simulink model "CM13_2024a_MachE_for_UA_HIL"  (R2024a)
settings: Solver=ode1  StartTime=0.0  StopTime=Inf  FixedStep=0.001  RelTol=1e-3  EnableMultiTasking=on
PreLoadFcn:
  | % if ~length(which('cmcmd')), cmenv; end
PostLoadFcn:
  | if any(exist('dsrtsu_mdlpostloadfcn', 'file') ~= 0), dsrtsu_mdlpostloadfcn('Execute', bdroot); end
InitFcn:
  | , if any(exist('rtifpga_mdlclblib', 'file') ~= 0), rtifpga_mdlclblib('Init', bdroot); end,
  | , if any(exist('dsmpb_private', 'file') ~= 0), dsmpb_private('dsmpb_mdlclblib', 'Init', bdroot); end,
values from neighbouring files (symbols this model uses):
  CoastDown =     [Run_Simulink.mat]
  limitedMCT =     [Run_Simulink.mat]
  MCT =     [Run_Simulink.mat]
  pMCT =     [Run_Simulink.mat]
  RealSimPara =     [Run_Simulink.mat]
  Ref_speed = [13 13.007895099 13.015778396 13.023649891 13.031509584 13.039357475 13.047193564 13.055017851 13.062830336 13.070631019 13.0784199 13.086196979 ... (2669 elements, 2669x1)]    [Ref_speed_and_time.mat]
  Ref_time = [0 0.01 0.02 0.03 0.04 0.05 0.06 0.07 0.08 0.09 0.1 0.11 ... (2669 elements, 2669x1)]    [Ref_speed_and_time.mat]
  US06 =     [Run_Simulink.mat]
undefined symbols (not defined in the file or in its folder): AccelCmd, ActTqLF_Nm_, ActTqLR_Nm_, ActTqRF_Nm_, ActTqRR_Nm_, BattChargeLimitMaxPwr, BattChargeLimitSocBpts, BattChargeLimitTbl, BattChrgCapcty, BattDischargeLimitSocBpts, BattDischargeLimitTbl, BattDischargeMaxPwr, BattNumCellsParallel, BattNumCellsSeries, BattOpenVoltCapBpts, BattOpenVoltTbl, BattResistSocBpts, BattResistTbl, BattResistTempBpts, BrakeMaxPrs, BrakeMaxTrq, ChassisDistCg2FrontAxle, ChassisDistCg2RearAxle, ChassisVehMass, CltchCmd, DecelCmd, DiffRatio, DiscIntNeverNeededParam, EnvGravCnst, EnvPrs, EnvTemp, FuelSpecificGrav, GearCmd, h, InitStates, lgSw, MtrEffSpdBpts, MtrEffTbl, MtrEffTrqBpts, MtrPwrMax, MtrTrqMax, planned_speed, planned_time, ref_speed, ref_time, rticanmm_blockfcn, rticanmm_initfcn, SteeringCmd, SupvsryCtrlRegenBrkCutOffTbl, SupvsryCtrlRegenSpdBpts, TestScnrioCycleNum, VEH
libraries: simulink x264, VSIGenLib x262, etargetslib x201, dsmpblib x161, CarMaker4SL x142, rtimmsu_dsrtlib x32, vehdynlibtire x24, autolibshared x19, vehdynlibsuspension x14, vehdynlibtirecommon x14, autolibutils x10, VsrLibWheel x8
(part 48 of 48)

== matlab function CM13_2024a_MachE_for_UA_HIL/RealSim1/MATLAB Function3 ==
  data: simState input; connectionState input; timeSimulator input; timeStepSimulator output; timeStepSimulatorPrevious input; timeStepTrigger output
function [timeStepSimulator, timeStepTrigger]  = fcn(simState, connectionState, timeSimulator, timeStepSimulatorPrevious)


if simState && abs(connectionState-3) < 1e-5 && (timeSimulator >= timeStepSimulatorPrevious + 0.1 - 1e-5 || abs(timeSimulator) < 1e-5)
    timeStepSimulator = timeSimulator;
    timeStepTrigger = 1;
else
    timeStepSimulator = timeStepSimulatorPrevious;
    timeStepTrigger = 0;
end

== matlab function CM13_2024a_MachE_for_UA_HIL/RealSim1/MATLAB Function4 ==
  data: simState input; simulatorStartTime output; simStatePrevious input; connectionState input; simulationTime input; simState output
function [simulatorStartTime, simState] = fcn(simState, simStatePrevious, connectionState, simulationTime)


if abs(simState - 1) < 1e-5 && abs(simStatePrevious) < 1e-5 && abs(connectionState-3) < 1e-5
    % set connectionState and start time
    simulatorStartTime = simulationTime;
else
    simulatorStartTime = 0;
end

== matlab function CM13_2024a_MachE_for_UA_HIL/FIXS1/RealSim Core/MATLAB Function1 ==
  data: obj input; simState output; ByteData input; nByte input; connectionState input; t output; nVeh output; VehDataBus output; isVehicleInNetwork output
function [simState, t, nVeh, VehDataBus, isVehicleInNetwork] = stepImpl(obj, ByteData, nByte, connectionState)

    simState = obj.simStatePrevious;
    t = obj.tPrevious;
    nVeh = 0;
    
    % init values for other variables
    totalMsgSize = 0; % this is the total message size received from Real-Sim
    msgProcessed = 0; % to record how many messages have been processed
    
    VehDataBus = obj.VehicleDataPrevious;

    %---------------------------
    % read received buffer
    %---------------------------
    % need to check size, before connection, there could be no
    % message at all             
    if nByte >= obj.msgHeaderSize
        simState = double(typecast(uint8(ByteData(1)),'uint8'));
        t = double(typecast(uint8(ByteData(2:5)),'single'));
        totalMsgSize = double(typecast(uint8(ByteData(6:9)),'uint32'));
        msgProcessed = obj.msgHeaderSize;
        
        obj.simStatePrevious = simState;
        obj.tPrevious = t;
    end
    
    % read actual message fields
    while round(msgProcessed) < round(totalMsgSize)
        iMsgSizeRecv = double(typecast(uint8(ByteData(msgProcessed+1:msgProcessed+2)),'uint16'));
        iMsgTypeRecv = double(typecast(uint8(ByteData(msgProcessed+3)),'uint8'));

        % !!! for now, Simulink only supports vehicle data type
        if obj.enableDebug
            obj.vehMsgIdentifer = iMsgTypeRecv;
        else
            obj.vehMsgIdentifer = 1;
        end
        
        if iMsgTypeRecv == obj.vehMsgIdentifer
            VehDataBus = obj.depackVehData(VehDataBus, ByteData(msgProcessed+obj.msgEachHeaderSize+1:msgProcessed+iMsgSizeRecv));
               
            nVeh = nVeh + 1;

            obj.VehicleDataPrevious = VehDataBus;
            obj.isVehicleInNetworkPrevious = 1;
        else
            % not supported yet!!!
            
        end
        
        msgProcessed = msgProcessed + iMsgSizeRecv;

    end
    

    if abs(connectionState-3)>1e-5
        % if not connected, then set to 0
        obj.simStatePrevious = 0;
        obj.tPrevious = 0;
        obj.nVehPrevious = 0;
        obj.VehicleDataPrevious = obj.VehicleDataEmpty;
        obj.isVehicleInNetworkPrevious = 0;
    else
        if totalMsgSize == 9
            obj.isVehicleInNetworkPrevious = 0;
        end
    end
    isVehicleInNetwork = obj.isVehicleInNetworkPrevious;

== matlab function CM13_2024a_MachE_for_UA_HIL/FIXS1/RealSim Core/generateTimeStepTrigger ==
  data: simState input; connectionState input; timeSimulation input; timeSimulationOut output; timeInOut output; timeSimulationPrevious input; timeStepTrigger output; timeIn input; timeInPrevious input
function [timeSimulationOut, timeInOut, timeStepTrigger]  = fcn(simState, connectionState, timeSimulation, timeSimulationPrevious, timeIn, timeInPrevious)


%if simState && abs(connectionState-3) < 1e-5 && (timeSimulator >= timeStepSimulatorPrevious + 0.1 - 1e-5 || abs(timeSimulator) < 1e-5)
% if simState && abs(connectionState-3) < 1e-5 && (timeSimulation >= timeSimulationPrevious + 0.1 - 1e-5)
if simState && abs(connectionState-3) < 1e-5 && ((timeSimulation >= timeSimulationPrevious + 0.1 - 1e-5) && (timeIn >= timeInPrevious + 0.1 - 1e-5))
    timeSimulationOut = timeSimulation;
    timeInOut = timeIn;
    timeStepTrigger = 1;
else
    timeSimulationOut = timeSimulationPrevious;
    timeInOut = timeInPrevious;
    timeStepTrigger = 0;
end

== matlab function CM13_2024a_MachE_for_UA_HIL/FIXS1/RealSim Translate CM Signal to Bus as Feedback to SUMO//VISSIM/MATLAB Function ==
  data: CM_POI_X input; positionX output; positionY output; positionZ output; heading output; color output; speedDesired output; CM_POI_Y input; CM_POI_Z input; CM_Fr1_X input; CM_Fr1_Y input; CM_Fr1_Z input; CM_yaw input; color_rgba input; CM_speed input
function [positionX, positionY, positionZ, heading, color, speedDesired] = ...
    RealSimSigTrans(CM_POI_X, CM_POI_Y, CM_POI_Z, CM_Fr1_X, CM_Fr1_Y, CM_Fr1_Z, CM_yaw, color_rgba, CM_speed)

% intialization
positionX = 0;
positionY = 0;
positionZ = 0;
heading = 0;
color = 0;
speedDesired = 0;

% convert position
% CM POI is CoM, CM Fr1 is back bottom of car
% SUMO-xy is front of car
% SUMO-z is bottom of car
positionX = CM_POI_X + (CM_POI_X - CM_Fr1_X);
positionY = CM_POI_Y + (CM_POI_Y - CM_Fr1_Y);
positionZ = CM_Fr1_Z;

% convert heading
if (CM_yaw >= -pi && CM_yaw <= 0.5 * pi)
    heading = ((-CM_yaw + 0.5 * pi) * 180 / pi);
else
    heading = ((-CM_yaw + 2.5 * pi) * 180 / pi);
end

% convert color from rgba to uint32
color = sum(color_rgba.*[2^24;2^16;2^8;2^0]);

% speed is same unit
speedDesired = CM_speed;

== stateflow chart CM13_2024a_MachE_for_UA_HIL/FIXS1/RealSimHILCycle ==
  state CycleOn
    state InitialWait
      CycleMode=1;
    state RampUp
      CycleMode=2;
      SpeedCmd=SpeedCmd+0.1
    state Driving
      CycleMode=3;
      SpeedCmd=max(SpeedIn, 0)
    state WaitForNextRamp
    InitialWait -> RampUp : [after(InitWaitTime,sec) || RampUpFlag]
    (default) -> InitialWait
    RampUp -> Driving [order 1] : [abs(SpeedCmd-SpeedInit)<0.5]
    RampUp -> CycleOn.WaitForNextRamp [order 2] : [abs(SpeedCmd-SpeedInit)>=0.1]
    CycleOn.WaitForNextRamp -> RampUp : after(0.1,sec)
  state Idle
    CycleMode=0;
    SpeedCmd=0;
    CycleTime=0;
  state RampDown
    CycleMode=4;
    SpeedCmd=SpeedCmd-1;
  state WaitForNextRamp
  (default) -> Idle
  Idle -> CycleOn : [SimState>=6 && ...
      | DistanceTravel <= totalDistance && ...
      | SimTime <= totalTime && ...
      | ~RampDownFlag]
  RampDown -> Idle [order 1] : [SpeedCmd<0.5]
  CycleOn -> RampDown : [DistanceTravel > totalDistance || ...
      | SimTime > totalTime || ...
      | RampDownFlag || ...
      | SimState==9]
  WaitForNextRamp -> RampDown : after(0.1,sec)
  RampDown -> WaitForNextRamp [order 2] : [SpeedCmd>=0.5]
  data: SimTime input; SimState input; SpeedIn input; DistanceTravel input; InitWaitTime input; SpeedInit input; totalDistance input; CycleMode output; SpeedCmd output; totalTime input; RampDownFlag input; CycleTime local; RampUpFlag input

== matlab function CM13_2024a_MachE_for_UA_HIL/RealSim2/MATLAB Function ==
  data: strUint8Vec input; intVal output double; strLen input
function intVal = strVec2Int(strUint8Vec, strLen)

    strVec = blanks(50);
    for i = 1:strLen
       strVec(i) = strUint8Vec(i); 
    end
    if strLen > 0
        intVal = real(str2double(strVec(1:strLen)));
    else
        intVal = -1;
    end

== matlab function CM13_2024a_MachE_for_UA_HIL/RealSim2/MATLAB Function1 ==
  data: strUint8Vec input; intVal output double; strLen input
function intVal = strVec2Int(strUint8Vec, strLen)

    strVec = blanks(50);
    for i = 1:strLen
       strVec(i) = strUint8Vec(i); 
    end
    if strLen > 0
        intVal = real(str2double(strVec(1:strLen)));
    else
        intVal = -1;
    end

== matlab function CM13_2024a_MachE_for_UA_HIL/RealSim2/MATLAB Function2 ==
  data: signalLightId input uint8 size=[1 50]; signalLightIdString output string; signalLightIdLength input
function signalLightIdString = fcn(signalLightId, signalLightIdLength)

signalLightIdString = string(char(signalLightId));

== matlab function CM13_2024a_MachE_for_UA_HIL/RealSim2/MATLAB Function3 ==
  data: simState input; connectionState input; timeSimulator input; timeStepSimulator output; timeStepSimulatorPrevious input; timeStepTrigger output
function [timeStepSimulator, timeStepTrigger]  = fcn(simState, connectionState, timeSimulator, timeStepSimulatorPrevious)


if simState && abs(connectionState-3) < 1e-5 && (timeSimulator >= timeStepSimulatorPrevious + 0.1 - 1e-5 || abs(timeSimulator) < 1e-5)
    timeStepSimulator = timeSimulator;
    timeStepTrigger = 1;
else
    timeStepSimulator = timeStepSimulatorPrevious;
    timeStepTrigger = 0;
end

== matlab function CM13_2024a_MachE_for_UA_HIL/RealSim2/MATLAB Function4 ==
  data: simState input; simulatorStartTime output; simStatePrevious input; connectionState input; simulationTime input; simState output
function [simulatorStartTime, simState] = fcn(simState, simStatePrevious, connectionState, simulationTime)


if abs(simState - 1) < 1e-5 && abs(simStatePrevious) < 1e-5 && abs(connectionState-3) < 1e-5
    % set connectionState and start time
    simulatorStartTime = simulationTime;
else
    simulatorStartTime = 0;
end

== stateflow chart CM13_2024a_MachE_for_UA_HIL/Vehicle Under Test2/Vehicle/Actuation and Outputs/MOOG Brake Actuator/MOOG Interface/MOOG State Machine ==
  state MainStateMachine [parallel]
    settings: executionOrder=2
    state Learning
      state LearnMinStop
        en:
        state BackStopCmd
          en:
          MoogOpMode=21 ;
          PositionCmd=-100000;
        state BackStopReached
          en:
          MoogOpMode=22;
          PositionCmd=0;
        state BackStopSettle
          en:
          MoogOpMode=23;
          MinStop=ActualPosition_cnt;
          PositionCmd=0;
        (default) -> MainStateMachine.Learning.LearnMinStop.BackStopCmd
        MainStateMachine.Learning.LearnMinStop.BackStopCmd -> MainStateMachine.Learning.LearnMinStop.BackStopReached : [bitand(StatusWord,8)]
        MainStateMachine.Learning.LearnMinStop.BackStopReached -> MainStateMachine.Learning.LearnMinStop.BackStopSettle : after(2,sec)
      state StartLearning
        en:
        MoogOpMode=11;
        PositionCmd=0;
        MinStop=-200000;
        MaxStop=200000;
      state LearnMaxStop
        en:
        state BackStopCmd
          en:
          MoogOpMode=31;
          PositionCmd=100000;
        state BackStopReached
          en:
          MoogOpMode=32;
          PositionCmd=0;
        state BackStopSettle
          en:
          MoogOpMode=33;
          MaxStop=ActualPosition_cnt;
          PositionCmd=0;
        (default) -> MainStateMachine.Learning.LearnMaxStop.BackStopCmd
        MainStateMachine.Learning.LearnMaxStop.BackStopCmd -> MainStateMachine.Learning.LearnMaxStop.BackStopReached : [bitand(StatusWord,8)]
        MainStateMachine.Learning.LearnMaxStop.BackStopReached -> MainStateMachine.Learning.LearnMaxStop.BackStopSettle : after(2,sec)
      state EndLearning
        en:
        MoogOpMode=41;
        PositionCmd=0;
        LearningComplete=1;
        FaultCntr=0;
      (default) -> StartLearning
      StartLearning -> LearnMinStop : after(0.5,sec)[InitComplete ==1]
      LearnMinStop -> LearnMaxStop : after(1,sec)[InitComplete ==1  && MinStop ~=-200000]
      LearnMaxStop -> EndLearning : after(1,sec)[InitComplete ==1  && MaxStop ~=200000 && ((MaxStop-MinStop)>ActuatorMinTravelForReady)]
    state NormalOperation
      state LearningNotComplete
        en:
        MoogOpMode=101;
        Actuator_Ready=0;
        du:
        PositionCmd=0;
      state LearningComplete
        en:
        MoogOpMode=102;
        Actuator_Ready=1;
        du:
        PositionCmd=TargetPosition_cnt;
      (default) -> LearningNotComplete
      LearningNotComplete -> LearningComplete : after(1,sec)[LearningComplete==1]
    MainStateMachine.Learning.LearnMaxStop.BackStopSettle -> NormalOperation : after(10,sec)
    Learning -> NormalOperation : after(1,sec)[LearningComplete==1]
    NormalOperation -> Learning : [PositionLearningTrigger==1]{Actuator_Ready =0;
        | LearningComplete=0}
    (default) -> NormalOperation : {Actuator_Ready =0;
        | LearningComplete=0}
  state MoogStateMachine [parallel]
    settings: executionOrder=1
    state Initialisation
      state SwitchOffDisabled
        % StatusWord= xxxx_xxxx_x0xx_0000, 0x00, 0d
        en:
        MoogSMState=13;
        ControlWord=0; % 0x00
      state Init
        en:
        MoogSMState=11;
        ControlWord=0;
        InitComplete =0;
      state ClearFault
        en:
        MoogSMState=12;
        ControlWord=128; % 0x80
      state SwitchOnDisabled
        % StatusWord= xxxx_xxxx_x1xx_0000, 0x40, 64d
        en:
        MoogSMState=14;
        ControlWord=6; % 0x06
      state ReadyToSwitchOn
        % StatusWord=xxxx_xxxx_x01x_0001, 0x21, 33d
        en:
        MoogSMState=15;
        ControlWord=7; % 0x07
      state SwitchedOn
        % StatusWord=xxxx_xxxx_x01x_0011, 0x23, 35d
        en:
        MoogSMState=16;
        ControlWord=15; % 0x0F
      state OperationEnabled
        % StatusWord=xxxx_xxxx_x01x_0111, 0x27, 39d
        en:
        MoogSMState=17;
        ControlWord=15; % 0x0F
        InitComplete=1;
      SwitchOffDisabled -> Init [order 2] : after(1,sec)[bitand(StatusWord,8)]{FaultCntr=FaultCntr+1;}
      (default) -> Init
      Init -> ClearFault : after(0.5,sec)
      ClearFault -> SwitchOffDisabled : after(0.5,sec)
      SwitchOffDisabled -> SwitchOnDisabled [order 1] : after(0.1,sec)[bitand(StatusWord,64)]
      OperationEnabled -> Init : after(1,sec)[bitand(StatusWord,8)]{FaultCntr=FaultCntr+1;}
      SwitchedOn -> Init [order 2] : after(1,sec)[bitand(StatusWord,8)]{FaultCntr=FaultCntr+1;}
      ReadyToSwitchOn -> Init [order 2] : after(1,sec)[bitand(StatusWord,8)]{FaultCntr=FaultCntr+1;}
      SwitchOnDisabled -> Init [order 2] : after(1,sec)[bitand(StatusWord,8)]{FaultCntr=FaultCntr+1;}
      SwitchOnDisabled -> ReadyToSwitchOn [order 1] : after(0.1,sec)[bitand(StatusWord,32) &...
          |  bitand(StatusWord,1)]
      ReadyToSwitchOn -> SwitchedOn [order 1] : after(0.1,sec)[bitand(StatusWord,32) & ...
          | bitand(StatusWord,2) & ...
          | bitand(StatusWord,1)]
      SwitchedOn -> OperationEnabled [order 1] : after(0.1,sec)[bitand(StatusWord,32) & ...
          | bitand(StatusWord,4) & ...
          | bitand(StatusWord,2) & ...
          | bitand(StatusWord,1)]
    state Wait
      en:
      MoogSMState=31;
      Actuator_Ready=0;
      InitComplete =0;
      LearningComplete=0;
    state PositionControl
      state EnableSetPoint
        en:
        MoogSMState=21;
        ControlWord=47; % 0x2F
      state BeginMotion
        en:
        MoogSMState=22;
        ControlWord=63; % 0x3F
      (default) -> EnableSetPoint
      EnableSetPoint -> BeginMotion : after(0.001,sec)[Actuator_Ready==1 || ...
          | MoogOpMode==21 || ...
          | MoogOpMode==31]
      BeginMotion -> EnableSetPoint : after(0.001,sec)
    Initialisation -> Wait [order 2] : after(2,sec)[CAN_CommsOK_Flg ==0]
    (default) -> Initialisation : {FaultCntr=0;}
    Initialisation -> Wait [order 3] : [FaultCntr>=5]
    Wait -> Initialisation : [ResetCmd &&CAN_CommsOK_Flg==1 ]{Actuator_Ready=0;FaultCntr=0;}
    Initialisation -> PositionControl [order 1] : [InitComplete==1]
    PositionControl -> Initialisation [order 1] : [ResetCmd ]{InitComplete=0;}
    PositionControl -> Initialisation [order 2] : [bitand(StatusWord,8)]{InitComplete=0;FaultCntr=FaultCntr+1;}
  data: CAN_CommsOK_Flg input; ControlWord output; PositionCmd output; ResetCmd input; PositionLearningTrigger input; StatusWord input; Actuator_Ready output; FaultCntr output; MoogSMState output; InitComplete output; MoogOpMode output; LearningComplete output; ActualPosition_cnt input; MaxStop output; MinStop output; TargetPosition_cnt input; ActuatorMinTravelForReady input

== matlab function CM13_2024a_MachE_for_UA_HIL/Vehicle Under Test2/Vehicle/Rototest and ORNL Interface/Get Wheel Spd Cmd Based on Wheel Dynamics/Whl Dynamics & Format CM Powertrain Signal/Subsystem/MATLAB Function ==
  data: axleTorq input; switchFlag output; wheelSpd input
function switchFlag = fcn(axleTorq, wheelSpd)

% if braking and vehicle has stopped
if (abs(axleTorq) < 1e-5 && abs(wheelSpd) < 1e-5)
    switchFlag = 1;
else
    switchFlag = 0;
end

== matlab function CM13_2024a_MachE_for_UA_HIL/Vehicle Under Test2/Vehicle/Rototest and ORNL Interface/Get Wheel Spd Cmd Based on Wheel Dynamics/Whl Dynamics & Format CM Powertrain Signal/Subsystem2/MATLAB Function ==
  data: axleTorq input; switchFlag output; wheelSpd input
function switchFlag = fcn(axleTorq, wheelSpd)

% if braking and vehicle has stopped
if (abs(axleTorq) < 1e-5 && abs(wheelSpd) < 1e-5)
    switchFlag = 1;
else
    switchFlag = 0;
end

== matlab function CM13_2024a_MachE_for_UA_HIL/Vehicle Under Test2/Vehicle/Rototest and ORNL Interface/Get Wheel Spd Cmd Based on Wheel Dynamics/Whl Dynamics & Format CM Powertrain Signal/Subsystem3/MATLAB Function ==
  data: axleTorq input; switchFlag output; wheelSpd input
function switchFlag = fcn(axleTorq, wheelSpd)

% if braking and vehicle has stopped
if (abs(axleTorq) < 1e-5 && abs(wheelSpd) < 1e-5)
    switchFlag = 1;
else
    switchFlag = 0;
end

== matlab function CM13_2024a_MachE_for_UA_HIL/Vehicle Under Test2/Vehicle/Rototest and ORNL Interface/Get Wheel Spd Cmd Based on Wheel Dynamics/Whl Dynamics & Format CM Powertrain Signal/Subsystem4/MATLAB Function ==
  data: axleTorq input; switchFlag output; wheelSpd input
function switchFlag = fcn(axleTorq, wheelSpd)

% if braking and vehicle has stopped
if (abs(axleTorq) < 1e-5 && abs(wheelSpd) < 1e-5)
    switchFlag = 1;
else
    switchFlag = 0;
end

== stateflow chart CM13_2024a_MachE_for_UA_HIL/Vehicle Under Test2/Vehicle/Rototest and ORNL Interface/To Rototest with Band-Aid/Band-Aid/Band-Aid ==
  state dStop
    en:
    OutMode = 0;
    State = 3;
  state Running
    state SpeedMode
      en:
      OutMode = 1;
      state Blend
        en:
        OutSpd = InSpd;
        State = 0.1;
      state Driving
        du:
        OutSpd = InSpd;
        State = 0.2;
      (default) -> Blend
      Blend -> Driving
    state TorqueMode
      en:
      OutMode = 0;
      du:
      State = 1;
    (default) -> SpeedMode
    TorqueMode -> Blend : [after(SettleTime, sec) || ...
        | ~BrkSw]
    SpeedMode -> TorqueMode : [(any(InSpd < SpdLatchThr) && ...
        | (VehSpd_kph < VehSpdThr_kph) && BrkSw)]
  note: The vehicle will enter speed mode (driving) if:
      | The vehicle has been in torque mode for a calibrated time (settleTime) AND
      | The Input Speed (InSpd) is greater than a Launch Treshold (LaunchSpdThr) OR
      | The Input Torque (InTrq) is greater than calibrated torque value (LaunchTrqThr).
      | Criteria 1) sees the dyno has "settled" and allows the dyno to go back into speed mode.
      | Criteria 2) sees the vehicle is attempting to reaccelerate and pushes into speed mode.
      |
      | The vehicle will enter torque mode (zero) if:
      | Input Speed (InSpd) goes below the calibrated speed (SpdLatchThr) AND
      | Brake (BrkSw) is active.
      | 2) dStop is activated.
      | Criteria 1) sees the vehicle is attempting to come to a stop and unloads the dyno.
      | Criteria 2) is SHTF.
      |
      | && ...
      | (InSpd > LaunchSpdThr || ...
      | InTrq > LaunchTrqThr)
  (default) -> dStop
  Running -> dStop : [dStop]
  dStop -> Running : [~dStop]
  data: LaunchSpdThr input; LaunchTrqThr input; SpdLatchThr input; BrkSw input; InSpd input; InTrq input; OutMode output size=1; OutSpd output; State output; SettleTime input; dStop input; VehSpd_kph input; VehSpdThr_kph input

== matlab function CM13_2024a_MachE_for_UA_HIL/Vehicle Under Test2/Vehicle/Rototest and ORNL Interface/To Rototest with Band-Aid/RotoTestEthTx/MATLAB Function ==
  data: SpTqRR input; y output; SpTqLR input; SpTqRF input; SpTqLF input; SystemActive input
function y = fcn(SpTqRR, SpTqLR, SpTqRF, SpTqLF, SystemActive)

y = 0;
if SpTqRR == 1 && SystemActive == 0
    y = 30;
elseif SpTqRR == 0 && SystemActive == 0
    y = 0;
elseif SpTqRR == 1 && SystemActive == 1
    y = 31;
elseif SpTqRR == 0 && SystemActive == 1
    y = 1;
end

y = uint8(y);

== matlab function CM13_2024a_MachE_for_UA_HIL/Vehicle Under Test2/Vehicle/Vehicle Dynamics/Vehicle 14DOF/Wheels and Tires/VDBS/Tires/MF Tires/MATLAB Function ==
  data: axleTorq input; switchFlag output; wheelSpd input
function switchFlag = fcn(axleTorq, wheelSpd)

% if braking and vehicle has stopped
%if (abs(axleTorq) < 1e-5 && abs(wheelSpd) < 1e-5)
if abs(wheelSpd) < 1e-5
    switchFlag = 1;
else
    switchFlag = 0;
end

== matlab function CM13_2024a_MachE_for_UA_HIL/Vehicle Under Test2/Vehicle/Vehicle Dynamics/Vehicle 14DOF/Wheels and Tires/VDBS/Tires/MF Tires/MATLAB Function1 ==
  data: axleTorq input; switchFlag output; wheelSpd input
function switchFlag = fcn(axleTorq, wheelSpd)

% if braking and vehicle has stopped
%if (abs(axleTorq) < 1e-5 && abs(wheelSpd) < 1e-5)
if abs(wheelSpd) < 1e-5
    switchFlag = 1;
else
    switchFlag = 0;
end

== matlab function CM13_2024a_MachE_for_UA_HIL/Vehicle Under Test2/Vehicle/Vehicle Dynamics/Vehicle 14DOF/Wheels and Tires/VDBS/Tires/MF Tires/MATLAB Function2 ==
  data: axleTorq input; switchFlag output; wheelSpd input
function switchFlag = fcn(axleTorq, wheelSpd)

% if braking and vehicle has stopped
%if (abs(axleTorq) < 1e-5 && abs(wheelSpd) < 1e-5)
if abs(wheelSpd) < 1e-5
    switchFlag = 1;
else
    switchFlag = 0;
end

== matlab function CM13_2024a_MachE_for_UA_HIL/Vehicle Under Test2/Vehicle/Vehicle Dynamics/Vehicle 14DOF/Wheels and Tires/VDBS/Tires/MF Tires/MATLAB Function3 ==
  data: axleTorq input; switchFlag output; wheelSpd input
function switchFlag = fcn(axleTorq, wheelSpd)

% if braking and vehicle has stopped
%if (abs(axleTorq) < 1e-5 && abs(wheelSpd) < 1e-5)
if abs(wheelSpd) < 1e-5
    switchFlag = 1;
else
    switchFlag = 0;
end

== matlab function CM13_2024a_MachE_for_UA_HIL/Vehicle Under Test2/Vehicle/Vehicle Dynamics/Vehicle 7DOF/For 3D Visualization ==
  data: angles output size=3; angleIn input size=3; GeomXYZ output size=3; GemoXYZIn input size=3; GroundZ input size=4; trackW parameter; wheelB parameter
function [angles,GeomXYZ]= three26(angleIn, GemoXYZIn, GroundZ,trackW, wheelB)%#codegen
coder.allowpcode('plain')
% Copyright 2018 The MathWorks, Inc.
[angles,GeomXYZ]= vdynthree2six(angleIn, GemoXYZIn, GroundZ,trackW, wheelB);

== stateflow chart CM13_2024a_MachE_for_UA_HIL/Vehicle Under Test3/Vehicle/Actuation and Outputs/MOOG Brake Actuator/MOOG Interface/MOOG State Machine ==
  state MainStateMachine [parallel]
    settings: executionOrder=2
    state Learning
      state LearnMinStop
        en:
        state BackStopCmd
          en:
          MoogOpMode=21 ;
          PositionCmd=-100000;
        state BackStopReached
          en:
          MoogOpMode=22;
          PositionCmd=0;
        state BackStopSettle
          en:
          MoogOpMode=23;
          MinStop=ActualPosition_cnt;
          PositionCmd=0;
        (default) -> MainStateMachine.Learning.LearnMinStop.BackStopCmd
        MainStateMachine.Learning.LearnMinStop.BackStopCmd -> MainStateMachine.Learning.LearnMinStop.BackStopReached : [bitand(StatusWord,8)]
        MainStateMachine.Learning.LearnMinStop.BackStopReached -> MainStateMachine.Learning.LearnMinStop.BackStopSettle : after(2,sec)
      state StartLearning
        en:
        MoogOpMode=11;
        PositionCmd=0;
        MinStop=-200000;
        MaxStop=200000;
      state LearnMaxStop
        en:
        state BackStopCmd
          en:
          MoogOpMode=31;
          PositionCmd=100000;
        state BackStopReached
          en:
          MoogOpMode=32;
          PositionCmd=0;
        state BackStopSettle
          en:
          MoogOpMode=33;
          MaxStop=ActualPosition_cnt;
          PositionCmd=0;
        (default) -> MainStateMachine.Learning.LearnMaxStop.BackStopCmd
        MainStateMachine.Learning.LearnMaxStop.BackStopCmd -> MainStateMachine.Learning.LearnMaxStop.BackStopReached : [bitand(StatusWord,8)]
        MainStateMachine.Learning.LearnMaxStop.BackStopReached -> MainStateMachine.Learning.LearnMaxStop.BackStopSettle : after(2,sec)
      state EndLearning
        en:
        MoogOpMode=41;
        PositionCmd=0;
        LearningComplete=1;
        FaultCntr=0;
      (default) -> StartLearning
      StartLearning -> LearnMinStop : after(0.5,sec)[InitComplete ==1]
      LearnMinStop -> LearnMaxStop : after(1,sec)[InitComplete ==1  && MinStop ~=-200000]
      LearnMaxStop -> EndLearning : after(1,sec)[InitComplete ==1  && MaxStop ~=200000 && ((MaxStop-MinStop)>ActuatorMinTravelForReady)]
    state NormalOperation
      state LearningNotComplete
        en:
        MoogOpMode=101;
        Actuator_Ready=0;
        du:
        PositionCmd=0;
      state LearningComplete
        en:
        MoogOpMode=102;
        Actuator_Ready=1;
        du:
        PositionCmd=TargetPosition_cnt;
      (default) -> LearningNotComplete
      LearningNotComplete -> LearningComplete : after(1,sec)[LearningComplete==1]
    MainStateMachine.Learning.LearnMaxStop.BackStopSettle -> NormalOperation : after(10,sec)
    Learning -> NormalOperation : after(1,sec)[LearningComplete==1]
    NormalOperation -> Learning : [PositionLearningTrigger==1]{Actuator_Ready =0;
        | LearningComplete=0}
    (default) -> NormalOperation : {Actuator_Ready =0;
        | LearningComplete=0}
  state MoogStateMachine [parallel]
    settings: executionOrder=1
    state Initialisation
      state SwitchOffDisabled
        % StatusWord= xxxx_xxxx_x0xx_0000, 0x00, 0d
        en:
        MoogSMState=13;
        ControlWord=0; % 0x00
      state Init
        en:
        MoogSMState=11;
        ControlWord=0;
        InitComplete =0;
      state ClearFault
        en:
        MoogSMState=12;
        ControlWord=128; % 0x80
      state SwitchOnDisabled
        % StatusWord= xxxx_xxxx_x1xx_0000, 0x40, 64d
        en:
        MoogSMState=14;
        ControlWord=6; % 0x06
      state ReadyToSwitchOn
        % StatusWord=xxxx_xxxx_x01x_0001, 0x21, 33d
        en:
        MoogSMState=15;
        ControlWord=7; % 0x07
      state SwitchedOn
        % StatusWord=xxxx_xxxx_x01x_0011, 0x23, 35d
        en:
        MoogSMState=16;
        ControlWord=15; % 0x0F
      state OperationEnabled
        % StatusWord=xxxx_xxxx_x01x_0111, 0x27, 39d
        en:
        MoogSMState=17;
        ControlWord=15; % 0x0F
        InitComplete=1;
      SwitchOffDisabled -> Init [order 2] : after(1,sec)[bitand(StatusWord,8)]{FaultCntr=FaultCntr+1;}
      (default) -> Init
      Init -> ClearFault : after(0.5,sec)
      ClearFault -> SwitchOffDisabled : after(0.5,sec)
      SwitchOffDisabled -> SwitchOnDisabled [order 1] : after(0.1,sec)[bitand(StatusWord,64)]
      OperationEnabled -> Init : after(1,sec)[bitand(StatusWord,8)]{FaultCntr=FaultCntr+1;}
      SwitchedOn -> Init [order 2] : after(1,sec)[bitand(StatusWord,8)]{FaultCntr=FaultCntr+1;}
      ReadyToSwitchOn -> Init [order 2] : after(1,sec)[bitand(StatusWord,8)]{FaultCntr=FaultCntr+1;}
      SwitchOnDisabled -> Init [order 2] : after(1,sec)[bitand(StatusWord,8)]{FaultCntr=FaultCntr+1;}
      SwitchOnDisabled -> ReadyToSwitchOn [order 1] : after(0.1,sec)[bitand(StatusWord,32) &...
          |  bitand(StatusWord,1)]
      ReadyToSwitchOn -> SwitchedOn [order 1] : after(0.1,sec)[bitand(StatusWord,32) & ...
          | bitand(StatusWord,2) & ...
          | bitand(StatusWord,1)]
      SwitchedOn -> OperationEnabled [order 1] : after(0.1,sec)[bitand(StatusWord,32) & ...
          | bitand(StatusWord,4) & ...
          | bitand(StatusWord,2) & ...
          | bitand(StatusWord,1)]
    state Wait
      en:
      MoogSMState=31;
      Actuator_Ready=0;
      InitComplete =0;
      LearningComplete=0;
    state PositionControl
      state EnableSetPoint
        en:
        MoogSMState=21;
        ControlWord=47; % 0x2F
      state BeginMotion
        en:
        MoogSMState=22;
        ControlWord=63; % 0x3F
      (default) -> EnableSetPoint
      EnableSetPoint -> BeginMotion : after(0.001,sec)[Actuator_Ready==1 || ...
          | MoogOpMode==21 || ...
          | MoogOpMode==31]
      BeginMotion -> EnableSetPoint : after(0.001,sec)
    Initialisation -> Wait [order 2] : after(2,sec)[CAN_CommsOK_Flg ==0]
    (default) -> Initialisation : {FaultCntr=0;}
    Initialisation -> Wait [order 3] : [FaultCntr>=5]
    Wait -> Initialisation : [ResetCmd &&CAN_CommsOK_Flg==1 ]{Actuator_Ready=0;FaultCntr=0;}
    Initialisation -> PositionControl [order 1] : [InitComplete==1]
    PositionControl -> Initialisation [order 1] : [ResetCmd ]{InitComplete=0;}
    PositionControl -> Initialisation [order 2] : [bitand(StatusWord,8)]{InitComplete=0;FaultCntr=FaultCntr+1;}
  data: CAN_CommsOK_Flg input; ControlWord output; PositionCmd output; ResetCmd input; PositionLearningTrigger input; StatusWord input; Actuator_Ready output; FaultCntr output; MoogSMState output; InitComplete output; MoogOpMode output; LearningComplete output; ActualPosition_cnt input; MaxStop output; MinStop output; TargetPosition_cnt input; ActuatorMinTravelForReady input

== matlab function CM13_2024a_MachE_for_UA_HIL/Vehicle Under Test3/Vehicle/Rototest and ORNL Interface/Get Wheel Spd Cmd Based on Wheel Dynamics/Whl Dynamics & Format CM Powertrain Signal/Subsystem/MATLAB Function ==
  data: axleTorq input; switchFlag output; wheelSpd input
function switchFlag = fcn(axleTorq, wheelSpd)

% if braking and vehicle has stopped
if (abs(axleTorq) < 1e-5 && abs(wheelSpd) < 1e-5)
    switchFlag = 1;
else
    switchFlag = 0;
end

== matlab function CM13_2024a_MachE_for_UA_HIL/Vehicle Under Test3/Vehicle/Rototest and ORNL Interface/Get Wheel Spd Cmd Based on Wheel Dynamics/Whl Dynamics & Format CM Powertrain Signal/Subsystem2/MATLAB Function ==
  data: axleTorq input; switchFlag output; wheelSpd input
function switchFlag = fcn(axleTorq, wheelSpd)

% if braking and vehicle has stopped
if (abs(axleTorq) < 1e-5 && abs(wheelSpd) < 1e-5)
    switchFlag = 1;
else
    switchFlag = 0;
end

== matlab function CM13_2024a_MachE_for_UA_HIL/Vehicle Under Test3/Vehicle/Rototest and ORNL Interface/Get Wheel Spd Cmd Based on Wheel Dynamics/Whl Dynamics & Format CM Powertrain Signal/Subsystem3/MATLAB Function ==
  data: axleTorq input; switchFlag output; wheelSpd input
function switchFlag = fcn(axleTorq, wheelSpd)

% if braking and vehicle has stopped
if (abs(axleTorq) < 1e-5 && abs(wheelSpd) < 1e-5)
    switchFlag = 1;
else
    switchFlag = 0;
end

== matlab function CM13_2024a_MachE_for_UA_HIL/Vehicle Under Test3/Vehicle/Rototest and ORNL Interface/Get Wheel Spd Cmd Based on Wheel Dynamics/Whl Dynamics & Format CM Powertrain Signal/Subsystem4/MATLAB Function ==
  data: axleTorq input; switchFlag output; wheelSpd input
function switchFlag = fcn(axleTorq, wheelSpd)

% if braking and vehicle has stopped
if (abs(axleTorq) < 1e-5 && abs(wheelSpd) < 1e-5)
    switchFlag = 1;
else
    switchFlag = 0;
end

== stateflow chart CM13_2024a_MachE_for_UA_HIL/Vehicle Under Test3/Vehicle/Rototest and ORNL Interface/To Rototest with Band-Aid/Band-Aid/Band-Aid ==
  state dStop
    en:
    OutMode = 0;
    State = 3;
  state Running
    state SpeedMode
      en:
      OutMode = 1;
      state Blend
        en:
        OutSpd = InSpd;
        State = 0.1;
      state Driving
        du:
        OutSpd = InSpd;
        State = 0.2;
      (default) -> Blend
      Blend -> Driving
    state TorqueMode
      en:
      OutMode = 0;
      du:
      State = 1;
    (default) -> SpeedMode
    TorqueMode -> Blend : [after(SettleTime, sec) || ...
        | ~BrkSw]
    SpeedMode -> TorqueMode : [(any(InSpd < SpdLatchThr) && ...
        | (VehSpd_kph < VehSpdThr_kph) && BrkSw)]
  note: The vehicle will enter speed mode (driving) if:
      | The vehicle has been in torque mode for a calibrated time (settleTime) AND
      | The Input Speed (InSpd) is greater than a Launch Treshold (LaunchSpdThr) OR
      | The Input Torque (InTrq) is greater than calibrated torque value (LaunchTrqThr).
      | Criteria 1) sees the dyno has "settled" and allows the dyno to go back into speed mode.
      | Criteria 2) sees the vehicle is attempting to reaccelerate and pushes into speed mode.
      |
      | The vehicle will enter torque mode (zero) if:
      | Input Speed (InSpd) goes below the calibrated speed (SpdLatchThr) AND
      | Brake (BrkSw) is active.
      | 2) dStop is activated.
      | Criteria 1) sees the vehicle is attempting to come to a stop and unloads the dyno.
      | Criteria 2) is SHTF.
      |
      | && ...
      | (InSpd > LaunchSpdThr || ...
      | InTrq > LaunchTrqThr)
  (default) -> dStop
  Running -> dStop : [dStop]
  dStop -> Running : [~dStop]
  data: LaunchSpdThr input; LaunchTrqThr input; SpdLatchThr input; BrkSw input; InSpd input; InTrq input; OutMode output size=1; OutSpd output; State output; SettleTime input; dStop input; VehSpd_kph input; VehSpdThr_kph input

== matlab function CM13_2024a_MachE_for_UA_HIL/Vehicle Under Test3/Vehicle/Rototest and ORNL Interface/To Rototest with Band-Aid/RotoTestEthTx/MATLAB Function ==
  data: SpTqRR input; y output; SpTqLR input; SpTqRF input; SpTqLF input; SystemActive input
function y = fcn(SpTqRR, SpTqLR, SpTqRF, SpTqLF, SystemActive)

y = 0;
if SpTqRR == 1 && SystemActive == 0
    y = 30;
elseif SpTqRR == 0 && SystemActive == 0
    y = 0;
elseif SpTqRR == 1 && SystemActive == 1
    y = 31;
elseif SpTqRR == 0 && SystemActive == 1
    y = 1;
end

y = uint8(y);

== matlab function CM13_2024a_MachE_for_UA_HIL/Vehicle Under Test3/Vehicle/Vehicle Dynamics/Vehicle 14DOF/Wheels and Tires/VDBS/Tires/MF Tires/MATLAB Function ==
  data: axleTorq input; switchFlag output; wheelSpd input
function switchFlag = fcn(axleTorq, wheelSpd)

% if braking and vehicle has stopped
%if (abs(axleTorq) < 1e-5 && abs(wheelSpd) < 1e-5)
if abs(wheelSpd) < 1e-5
    switchFlag = 1;
else
    switchFlag = 0;
end

== matlab function CM13_2024a_MachE_for_UA_HIL/Vehicle Under Test3/Vehicle/Vehicle Dynamics/Vehicle 14DOF/Wheels and Tires/VDBS/Tires/MF Tires/MATLAB Function1 ==
  data: axleTorq input; switchFlag output; wheelSpd input
function switchFlag = fcn(axleTorq, wheelSpd)

% if braking and vehicle has stopped
%if (abs(axleTorq) < 1e-5 && abs(wheelSpd) < 1e-5)
if abs(wheelSpd) < 1e-5
    switchFlag = 1;
else
    switchFlag = 0;
end

== matlab function CM13_2024a_MachE_for_UA_HIL/Vehicle Under Test3/Vehicle/Vehicle Dynamics/Vehicle 14DOF/Wheels and Tires/VDBS/Tires/MF Tires/MATLAB Function2 ==
  data: axleTorq input; switchFlag output; wheelSpd input
function switchFlag = fcn(axleTorq, wheelSpd)

% if braking and vehicle has stopped
%if (abs(axleTorq) < 1e-5 && abs(wheelSpd) < 1e-5)
if abs(wheelSpd) < 1e-5
    switchFlag = 1;
else
    switchFlag = 0;
end

== matlab function CM13_2024a_MachE_for_UA_HIL/Vehicle Under Test3/Vehicle/Vehicle Dynamics/Vehicle 14DOF/Wheels and Tires/VDBS/Tires/MF Tires/MATLAB Function3 ==
  data: axleTorq input; switchFlag output; wheelSpd input
function switchFlag = fcn(axleTorq, wheelSpd)

% if braking and vehicle has stopped
%if (abs(axleTorq) < 1e-5 && abs(wheelSpd) < 1e-5)
if abs(wheelSpd) < 1e-5
    switchFlag = 1;
else
    switchFlag = 0;
end

== matlab function CM13_2024a_MachE_for_UA_HIL/Vehicle Under Test3/Vehicle/Vehicle Dynamics/Vehicle 7DOF/For 3D Visualization ==
  data: angles output size=3; angleIn input size=3; GeomXYZ output size=3; GemoXYZIn input size=3; GroundZ input size=4; trackW parameter; wheelB parameter
function [angles,GeomXYZ]= three26(angleIn, GemoXYZIn, GroundZ,trackW, wheelB)%#codegen
coder.allowpcode('plain')
% Copyright 2018 The MathWorks, Inc.
[angles,GeomXYZ]= vdynthree2six(angleIn, GemoXYZIn, GroundZ,trackW, wheelB);

== stateflow chart CM13_2024a_MachE_for_UA_HIL/CarMaker_new/IPG Vehicle/Actuation and Outputs/MOOG Brake Actuator/MOOG Interface/MOOG State Machine ==
  state MainStateMachine [parallel]
    settings: executionOrder=2
    state Learning
      state LearnMinStop
        en:
        state BackStopCmd
          en:
          MoogOpMode=21 ;
          PositionCmd=-100000;
        state BackStopReached
          en:
          MoogOpMode=22;
          PositionCmd=0;
        state BackStopSettle
          en:
          MoogOpMode=23;
          MinStop=ActualPosition_cnt;
          PositionCmd=0;
        (default) -> MainStateMachine.Learning.LearnMinStop.BackStopCmd
        MainStateMachine.Learning.LearnMinStop.BackStopCmd -> MainStateMachine.Learning.LearnMinStop.BackStopReached : [bitand(StatusWord,8)]
        MainStateMachine.Learning.LearnMinStop.BackStopReached -> MainStateMachine.Learning.LearnMinStop.BackStopSettle : after(2,sec)
      state StartLearning
        en:
        MoogOpMode=11;
        PositionCmd=0;
        MinStop=-200000;
        MaxStop=200000;
      state LearnMaxStop
        en:
        state BackStopCmd
          en:
          MoogOpMode=31;
          PositionCmd=100000;
        state BackStopReached
          en:
          MoogOpMode=32;
          PositionCmd=0;
        state BackStopSettle
          en:
          MoogOpMode=33;
          MaxStop=ActualPosition_cnt;
          PositionCmd=0;
        (default) -> MainStateMachine.Learning.LearnMaxStop.BackStopCmd
        MainStateMachine.Learning.LearnMaxStop.BackStopCmd -> MainStateMachine.Learning.LearnMaxStop.BackStopReached : [bitand(StatusWord,8)]
        MainStateMachine.Learning.LearnMaxStop.BackStopReached -> MainStateMachine.Learning.LearnMaxStop.BackStopSettle : after(2,sec)
      state EndLearning
        en:
        MoogOpMode=41;
        PositionCmd=0;
        LearningComplete=1;
        FaultCntr=0;
      (default) -> StartLearning
      StartLearning -> LearnMinStop : after(0.5,sec)[InitComplete ==1]
      LearnMinStop -> LearnMaxStop : after(1,sec)[InitComplete ==1  && MinStop ~=-200000]
      LearnMaxStop -> EndLearning : after(1,sec)[InitComplete ==1  && MaxStop ~=200000 && ((MaxStop-MinStop)>ActuatorMinTravelForReady)]
    state NormalOperation
      state LearningNotComplete
        en:
        MoogOpMode=101;
        Actuator_Ready=0;
        du:
        PositionCmd=0;
      state LearningComplete
        en:
        MoogOpMode=102;
        Actuator_Ready=1;
        du:
        PositionCmd=TargetPosition_cnt;
      (default) -> LearningNotComplete
      LearningNotComplete -> LearningComplete : after(1,sec)[LearningComplete==1]
    MainStateMachine.Learning.LearnMaxStop.BackStopSettle -> NormalOperation : after(10,sec)
    Learning -> NormalOperation : after(1,sec)[LearningComplete==1]
    NormalOperation -> Learning : [PositionLearningTrigger==1]{Actuator_Ready =0;
        | LearningComplete=0}
    (default) -> NormalOperation : {Actuator_Ready =0;
        | LearningComplete=0}
  state MoogStateMachine [parallel]
    settings: executionOrder=1
    state Initialisation
      state SwitchOffDisabled
        % StatusWord= xxxx_xxxx_x0xx_0000, 0x00, 0d
        en:
        MoogSMState=13;
        ControlWord=0; % 0x00
      state Init
        en:
        MoogSMState=11;
        ControlWord=0;
        InitComplete =0;
      state ClearFault
        en:
        MoogSMState=12;
        ControlWord=128; % 0x80
      state SwitchOnDisabled
        % StatusWord= xxxx_xxxx_x1xx_0000, 0x40, 64d
        en:
        MoogSMState=14;
        ControlWord=6; % 0x06
      state ReadyToSwitchOn
        % StatusWord=xxxx_xxxx_x01x_0001, 0x21, 33d
        en:
        MoogSMState=15;
        ControlWord=7; % 0x07
      state SwitchedOn
        % StatusWord=xxxx_xxxx_x01x_0011, 0x23, 35d
        en:
        MoogSMState=16;
        ControlWord=15; % 0x0F
      state OperationEnabled
        % StatusWord=xxxx_xxxx_x01x_0111, 0x27, 39d
        en:
        MoogSMState=17;
        ControlWord=15; % 0x0F
        InitComplete=1;
      SwitchOffDisabled -> Init [order 2] : after(1,sec)[bitand(StatusWord,8)]{FaultCntr=FaultCntr+1;}
      (default) -> Init
      Init -> ClearFault : after(0.5,sec)
      ClearFault -> SwitchOffDisabled : after(0.5,sec)
      SwitchOffDisabled -> SwitchOnDisabled [order 1] : after(0.1,sec)[bitand(StatusWord,64)]
      OperationEnabled -> Init : after(1,sec)[bitand(StatusWord,8)]{FaultCntr=FaultCntr+1;}
      SwitchedOn -> Init [order 2] : after(1,sec)[bitand(StatusWord,8)]{FaultCntr=FaultCntr+1;}
      ReadyToSwitchOn -> Init [order 2] : after(1,sec)[bitand(StatusWord,8)]{FaultCntr=FaultCntr+1;}
      SwitchOnDisabled -> Init [order 2] : after(1,sec)[bitand(StatusWord,8)]{FaultCntr=FaultCntr+1;}
      SwitchOnDisabled -> ReadyToSwitchOn [order 1] : after(0.1,sec)[bitand(StatusWord,32) &...
          |  bitand(StatusWord,1)]
      ReadyToSwitchOn -> SwitchedOn [order 1] : after(0.1,sec)[bitand(StatusWord,32) & ...
          | bitand(StatusWord,2) & ...
          | bitand(StatusWord,1)]
      SwitchedOn -> OperationEnabled [order 1] : after(0.1,sec)[bitand(StatusWord,32) & ...
          | bitand(StatusWord,4) & ...
          | bitand(StatusWord,2) & ...
          | bitand(StatusWord,1)]
    state Wait
      en:
      MoogSMState=31;
      Actuator_Ready=0;
      InitComplete =0;
      LearningComplete=0;
    state PositionControl
      state EnableSetPoint
        en:
        MoogSMState=21;
        ControlWord=47; % 0x2F
      state BeginMotion
        en:
        MoogSMState=22;
        ControlWord=63; % 0x3F
      (default) -> EnableSetPoint
      EnableSetPoint -> BeginMotion : after(0.001,sec)[Actuator_Ready==1 || ...
          | MoogOpMode==21 || ...
          | MoogOpMode==31]
      BeginMotion -> EnableSetPoint : after(0.001,sec)
    Initialisation -> Wait [order 2] : after(2,sec)[CAN_CommsOK_Flg ==0]
    (default) -> Initialisation : {FaultCntr=0;}
    Initialisation -> Wait [order 3] : [FaultCntr>=5]
    Wait -> Initialisation : [ResetCmd &&CAN_CommsOK_Flg==1 ]{Actuator_Ready=0;FaultCntr=0;}
    Initialisation -> PositionControl [order 1] : [InitComplete==1]
    PositionControl -> Initialisation [order 1] : [ResetCmd ]{InitComplete=0;}
    PositionControl -> Initialisation [order 2] : [bitand(StatusWord,8)]{InitComplete=0;FaultCntr=FaultCntr+1;}
  data: CAN_CommsOK_Flg input; ControlWord output; PositionCmd output; ResetCmd input; PositionLearningTrigger input; StatusWord input; Actuator_Ready output; FaultCntr output; MoogSMState output; InitComplete output; MoogOpMode output; LearningComplete output; ActualPosition_cnt input; MaxStop output; MinStop output; TargetPosition_cnt input; ActuatorMinTravelForReady input
